simulink model "lidarBus"  (R2022b)
settings: Solver=FixedStepAuto  StartTime=0.0  StopTime=inf  FixedStep=0.01  RelTol=1e-3  EnableMultiTasking=on
InitFcn:
  | Ts = 0.01;
model workspace (MAT data in the model file):
  SL_ROS_VariableLengthArrays_MaxSizes.CommonInfo.ArrayTruncateAction = 'EmitWarning'
  SL_ROS_VariableLengthArrays_MaxSizes.MsgTypeMap = containers.Map
  SL_ROS_VariableLengthArrays_MaxSizes.MsgTypeMap.serialization.keys = {'sensor_msgs/LaserScan', 'std_msgs/Header'}
  SL_ROS_VariableLengthArrays_MaxSizes.MsgTypeMap.serialization.values{1}(1).PropertyName = 'intensities'
  SL_ROS_VariableLengthArrays_MaxSizes.MsgTypeMap.serialization.values{1}(1).DataType = 'single'
  SL_ROS_VariableLengthArrays_MaxSizes.MsgTypeMap.serialization.values{1}(1).MaxLength = 40
  SL_ROS_VariableLengthArrays_MaxSizes.MsgTypeMap.serialization.values{1}(2).PropertyName = 'ranges'
  SL_ROS_VariableLengthArrays_MaxSizes.MsgTypeMap.serialization.values{1}(2).DataType = 'single'
  SL_ROS_VariableLengthArrays_MaxSizes.MsgTypeMap.serialization.values{1}(2).MaxLength = 40
  SL_ROS_VariableLengthArrays_MaxSizes.MsgTypeMap.serialization.values{2}.PropertyName = 'frame_id'
  SL_ROS_VariableLengthArrays_MaxSizes.MsgTypeMap.serialization.values{2}.DataType = 'uint8'
  SL_ROS_VariableLengthArrays_MaxSizes.MsgTypeMap.serialization.values{2}.MaxLength = 11
  SL_ROS_VariableLengthArrays_MaxSizes.MsgTypeMap.serialization.uniformity = 0
  SL_ROS_VariableLengthArrays_MaxSizes.MsgTypeMap.serialization.keyType = 'char'
  SL_ROS_VariableLengthArrays_MaxSizes.MsgTypeMap.serialization.valueType = 'any'
libraries: ros2lib x3, instrumentseriallib x2
settings Model: Creator=System-10  LastModifiedBy=System-10
settings SolverCC: PositivePriorityOrder=on
settings OptimizationCC: EnhancedBackFolding=on  PassReuseOutputArgsAs=Individual arguments  ZeroExternalMemoryAtStartup=off  ZeroInternalMemoryAtStartup=off  MaxStackSize=64  OptimizeBlockOrder=speed  DifferentSizesBufferReuse=on  OptimizationCustomize=off  EfficientTunableParamExpr=on
settings DebuggingCC: ParameterTunabilityLossMsg=error
settings HardwareCC: ProdBitPerPointer=32  ProdBitPerSizeT=32  ProdBitPerPtrDiffT=32  ProdLargestAtomicInteger=Long  ProdLargestAtomicFloat=Double  ProdWordSize=32  ProdHWDeviceType=ARM Compatible->ARM Cortex
settings ModelReferenceCC: ModelReferenceNumInstancesAllowed=Single  PropagateVarSize=During execution
settings RTWCC: Description=Embedded Coder  SystemTargetFile=ert.tlc  HardwareBoard=Raspberry Pi - Robot Operating System (ROS)  TLCOptions="-aInlineSetEventsForThisBaseRateFcn=TLC_FALSE -aSuppressMultiTaskScheduler=TLC_FALSE    -aRateBasedStepFcn=0"  TemplateMakefile=ert_default_tmf  Toolchain=Catkin  BuildConfiguration=Faster Runs  TargetLang=C++
settings CodeAppCC: ForceParamTrailComments=on  IgnoreCustomStorageClasses=off  OperatorAnnotations=on  SimulinkDataObjDesc=on  SFDataObjDesc=on  InsertBlockDesc=on
settings ERTTargetCC: SupportVariableSizeSignals=on  RootIOFormat=Structure reference

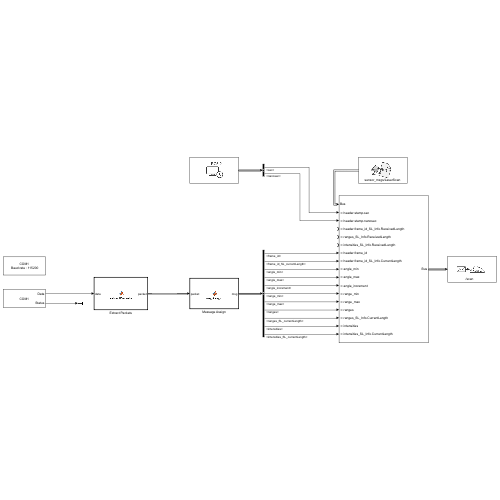
[thumbnail: Simulink's stored preview of the top-level diagram]
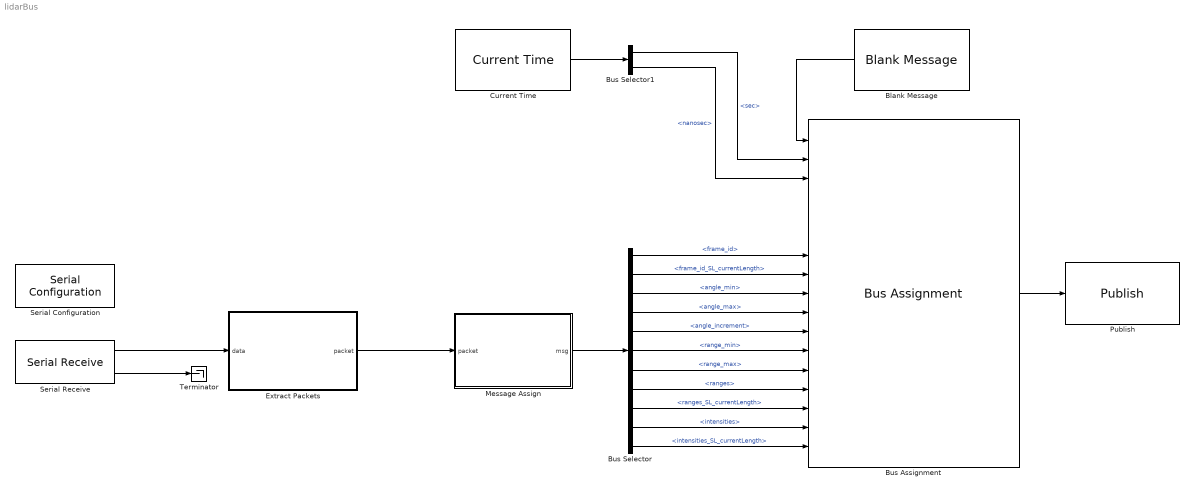
== system lidarBus ==
  Blank Message : ros2lib/Blank Message  messageClass=Message  entityType=sensor_msgs/LaserScan  messageType=sensor_msgs/LaserScan  SampleTime=Ts
      settings: LibrarySourceBlock=roslib/ROS 2/Blank Message
  Bus Assignment : BusAssignment  AssignedSignals=header.stamp.sec,header.stamp.nanosec,header.frame_id_SL_Info.ReceivedLength,ranges_SL_Info.ReceivedLength,intensities_SL_Info.ReceivedLength,header.frame_id,header.frame_id_SL_Info.CurrentLength,angle_min,angle_max,angle_increment,range_min,range_max,ranges,ranges_SL_Info.CurrentLength,intensities,intensities_SL_Info.CurrentLength
  Bus Selector : BusSelector  OutputSignals=header.frame_id,header.frame_id_SL_currentLength,angle_min,angle_max,angle_increment,range_min,range_max,ranges,ranges_SL_currentLength,intensities,intensities_SL_currentLength
  Bus Selector1 : BusSelector  OutputSignals=sec,nanosec
  Current Time : ros2lib/Current Time  OutputFormat=bus  SampleTime=Ts  ModelName=lidarBus
      settings: LibrarySourceBlock=roslib/ROS 2/Current Time
  Extract Packets : MATLAB Function  TreatAsAtomicUnit=on
  Message Assign : MATLAB Function  TreatAsAtomicUnit=on
  Publish : ros2lib/Publish  topicSource=Specify your own  topic=/scan  messageType=sensor_msgs/LaserScan  QOSHistory=Keep last  QOSDepth=1  QOSReliability=Reliable  QOSDurability=Volatile
      settings: LibrarySourceBlock=roslib/ROS 2/Publish
  Serial Configuration : instrumentseriallib/Serial Configuration  Priority=-200000  PortSel=COM1  Port=COM1  ComPort=COM1  BaudRate=115200  DataBits=8  Parity=none  StopBits=1  ByteOrder=little-endian  FlowControl=none  Timeout=10  SimulateUsing=Interpreted execution  BlockInModel=on  aMode=1
  Serial Receive : instrumentseriallib/Serial Receive  Priority=1  PortSel=COM1  Port=COM1  ComPort=COM1  DataType=uint8  SaveDataType=uint8  ToggleHeader=off  Header=[170 85]  ToggleTerminator=off  Terminator=<none>  CustomTerminator=[]  InputFormat=Column major  ToggleDataSize=on  DataSize=[1 2000]  EnableBlockingMode=off  ActionDataUnavailable=Output last received value  ActionWhenDataUnavailable=Output last received value  CustomValue=111  SampleTime=Ts  SimulateUsing=Interpreted execution  BlockInModel=on  aMode=1
  Terminator : Terminator
  wires:
  Message Assign/1(msg) -> Bus Selector/1
  Blank Message/1 -> Bus Assignment/1
  Current Time/1 -> Bus Selector1/1
  Bus Selector1/1 -> Bus Assignment/2  "<sec>"
  Bus Selector1/2 -> Bus Assignment/3  "<nanosec>"
  Bus Selector/1 -> Bus Assignment/7  "<frame_id>"
  Bus Selector/3 -> Bus Assignment/9  "<angle_min>"
  Bus Selector/4 -> Bus Assignment/10  "<angle_max>"
  Bus Selector/5 -> Bus Assignment/11  "<angle_increment>"
  Bus Selector/6 -> Bus Assignment/12  "<range_min>"
  Bus Selector/7 -> Bus Assignment/13  "<range_max>"
  Bus Selector/8 -> Bus Assignment/14  "<ranges>"
  Bus Selector/10 -> Bus Assignment/16  "<intensities>"
  Bus Assignment/1 -> Publish/1
  Bus Selector/2 -> Bus Assignment/8  "<frame_id_SL_currentLength>"
  Bus Selector/9 -> Bus Assignment/15  "<ranges_SL_currentLength>"
  Bus Selector/11 -> Bus Assignment/17  "<intensities_SL_currentLength>"
  Extract Packets/1(packet) -> Message Assign/1(packet)
  Serial Receive/2 -> Terminator/1
  Serial Receive/1 -> Extract Packets/1(data)

== matlab function lidarBus/Extract Packets ==
  settings: updateMethod=DISCRETE  sampleTime=Ts
  data: data input; packet output double size=[100 100]
function packet = extractPackets(data)
    
    data  = data';
    persistent indicesOfHeaders;
    persistent startIdx;
    persistent endIdx;
    persistent idx;
    persistent lastData;

    if isempty(lastData)
        lastData = uint8(zeros(1,size(data,2)));
    end

    if isempty(indicesOfHeaders) || ~isequal(data, lastData)
        
        indicesOfAA = find(data == 170);
        indicesOfHeaders = zeros(1, length(indicesOfAA)); 
        count = 0;
        
        startIdx = 0;
        endIdx = 0;
        idx = 0;

        for i = 1:length(indicesOfAA)
            if indicesOfAA(i) < length(data) && data(indicesOfAA(i) + 1) == 85
                count = count + 1;
                indicesOfHeaders(count) = indicesOfAA(i);
            end
        end

        indicesOfHeaders = indicesOfHeaders(1:count);
        lastData = data;      
    end
    
    if endIdx < indicesOfHeaders(end)
        idx = idx + 1;
        startIdx = indicesOfHeaders(idx);
        endIdx = indicesOfHeaders(idx+1);
        packet = double(data(startIdx:endIdx-1));
    else
        packet = [];
    end
end

== matlab function lidarBus/Message Assign ==
  settings: updateMethod=DISCRETE  sampleTime=Ts
  data: msg output Bus: std_msgs_LaserScan; packet input
function msg = msgAssign(packet)
    
    msg.header.frame_id = uint8([108, 105, 100, 97, 114, 95, 102, 114, 97, 109, 101]);
    msg.header.frame_id_SL_currentLength = uint32(length(msg.header.frame_id));
    msg.angle_min = single(1);
    msg.angle_max = single(2);
    msg.angle_increment = single(1);
    msg.range_min = single(0.1);
    msg.range_max = single(8);
    msg.ranges = single(ones(1,40));
    msg.ranges_SL_currentLength = uint32(size(msg.ranges,2));
    msg.intensities = single(zeros(1,40));
    msg.intensities_SL_currentLength = uint32(size(msg.intensities,2));

    if size(packet, 2) < 90
       msg.ranges_SL_currentLength = uint32(0);
       msg.intensities_SL_currentLength = uint32(0);
       return;
    end
        
    LSN = packet(1, 4);
    FSA = double(bitor(bitshift(uint16(packet(1, 6)), 8), uint16(packet(1, 5)), 'uint16'));
    LSA = double(bitor(bitshift(uint16(packet(1, 8)), 8), uint16(packet(1, 7)), 'uint16'));

    AngleFSA = double(bitshift(FSA, -1) / 64);
        msg.angle_min = single(deg2rad(AngleFSA));
    AngleLSA = double(bitshift(LSA, -1) / 64);
        msg.angle_max = single(deg2rad(AngleLSA));
    diffAngle = mod((AngleLSA - AngleFSA),360);
        msg.angle_increment = single(deg2rad(diffAngle)/LSN);
            
    rawSi = uint8(packet(:, 11:end));
    Si = zeros(1, 40);
    for i = 1:2:length(rawSi)
       Si((i + 1) / 2) = double(bitor(bitshift(uint16(rawSi(1, i + 1)), 8), uint16(rawSi(1, i)), 'uint16'));
    end
    Si = Si / 4000;
    msg.ranges = single(Si);
    
end
